simulink model "Lese_GPS_posisjon"  (R2018a)
settings: Solver=FixedStepAuto  StartTime=0.0  StopTime=inf  RelTol=1e-3  EnableMultiTasking=on
libraries: arduinolib x1
settings Model: SimulationMode=external  ExtModeTrigDuration=2  Creator=The MathWorks, Inc.  LastModifiedBy=halva
settings DataIOCC: LimitDataPoints=on
settings OptimizationCC: LifeSpan=Inf  MaxStackSize=64
settings DebuggingCC: AllowSymbolicDim=off  SFUnexpectedBacktrackingDiag=warning  SFNoUnconditionalDefaultTransitionDiag=warning  SFExecutionAtInitializationDiag=none
settings HardwareCC: ProdBitPerInt=16  ProdBitPerPointer=16  ProdBitPerSizeT=16  ProdBitPerPtrDiffT=16  ProdLargestAtomicFloat=None  ProdWordSize=8  ProdHWDeviceType=Atmel->AVR  UseEmbeddedCoderFeatures=off  UseSimulinkCoderFeatures=off
settings ModelReferenceCC: PropagateSignalLabelsOutOfModel=off
settings SFSimCC: MATLABDynamicMemAlloc=off
settings RTWCC: SystemTargetFile=ert.tlc  HardwareBoard=Arduino Mega 2560  TemplateMakefile=ert_default_tmf  Toolchain=Arduino AVR  BuildConfiguration=Faster Runs
settings CodeAppCC: MangleLength=10  StateflowObjectComments=on
settings ERTTargetCC: MultiwordLength=2048  ERTCustomFileBanners=off  SupportContinuousTime=on  SupportNonInlinedSFcns=on  RemoveResetFunc=off  ModelStepFunctionPrototypeControlCompliant=off  ConvertIfToSwitch=off  SuppressUnreachableDefaultCases=off
settings ConfigComp: CovMetricSettings=dw  CovHtmlReporting=on  CovSaveCumulativeToWorkspaceVar=on  CovSaveSingleToWorkspaceVar=on  CovExternalEMLEnable=off

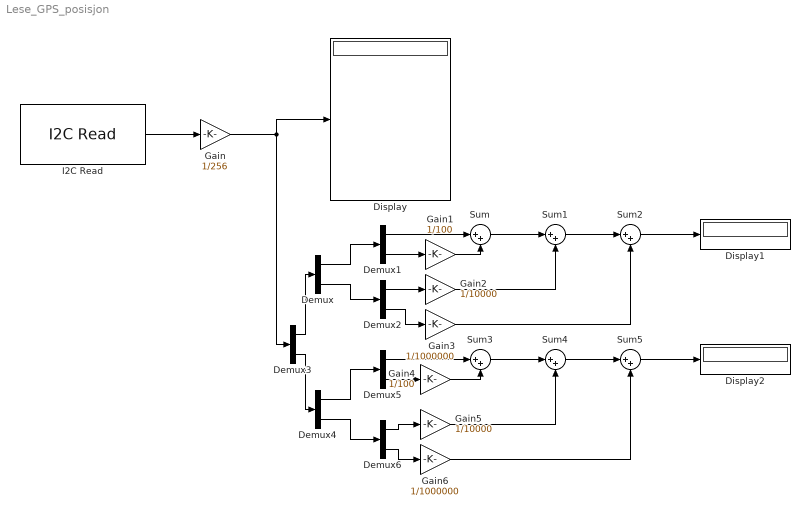
== system Lese_GPS_posisjon ==
  Demux{,1..6} (7 alike) : Demux  Outputs=2
  Display : Display
  Display1 : Display
      settings: Format=decimal (Stored Integer)
  Display2 : Display
      settings: Format=decimal (Stored Integer)
  Gain : Gain  Gain=1/256  OutDataTypeStr=double
  Gain1 : Gain  Gain=1/100
  Gain2 : Gain  Gain=1/10000
  Gain3 : Gain  Gain=1/1000000
  Gain4 : Gain  Gain=1/100
  Gain5 : Gain  Gain=1/10000
  Gain6 : Gain  Gain=1/1000000
  I2C Read : arduinolib/I2C Read  SlaveAddress_=hex2dec( '48' )  RegisterAddressEnable=off  RegisterAddress_=hex2dec( '20' )  Datatype=uint16  ByteOrder=Big Endian  Datalength_=8  SampleTime_=0.5  blockPlatform=arduino
      settings: SourceProductName=Simulink Support Package for Arduino Hardware  SourceProductBaseCode=ARDUINO
  Sum{,1..5} (6 alike) : Sum  Inputs=|++
  wires:
  I2C Read/1 -> Gain/1
  Demux/2 -> Demux2/1
  Demux/1 -> Demux1/1
  Demux1/2 -> Gain1/1
  Demux1/1 -> Sum/1
  Gain1/1 -> Sum/2
  Demux2/1 -> Gain2/1
  Gain2/1 -> Sum1/2
  Sum/1 -> Sum1/1
  Demux2/2 -> Gain3/1
  Gain3/1 -> Sum2/2
  Sum1/1 -> Sum2/1
  Sum2/1 -> Display1/1
  Gain/1 -> Demux3/1, Display/1
  Demux4/1 -> Demux5/1
  Demux4/2 -> Demux6/1
  Demux5/2 -> Gain4/1
  Demux6/1 -> Gain5/1
  Demux6/2 -> Gain6/1
  Demux5/1 -> Sum3/1
  Sum3/1 -> Sum4/1
  Sum4/1 -> Sum5/1
  Gain4/1 -> Sum3/2
  Gain5/1 -> Sum4/2
  Gain6/1 -> Sum5/2
  Sum5/1 -> Display2/1
  Demux3/1 -> Demux/1
  Demux3/2 -> Demux4/1
